simulink model "Simulation_2Sensors"  (R2020a)
settings: Solver=VariableStepAuto  StartTime=0.0  StopTime=18  RelTol=1e-3
values from neighbouring files (symbols this model uses):
  Pixels = [0 0 0 0 0 0 0 0 0 0 0 0 ... (1000000 elements, 1000x1000)]    [CrossMap.mat]    (also in GenerateCourseData.m = zeros(Height, Width); Pixels.mat = [0 0 0 0 0 0 0 0 0 0 0 0 ... (19600 elements, 140x140)])
  scale = 1    [GenerateCourseData.m]
undefined symbols (not defined in the file or in its folder): DiscIntNeverNeededParam, l, sensRange, w
libraries: simulink x1
settings Model: Creator=robot  LastModifiedBy=robot

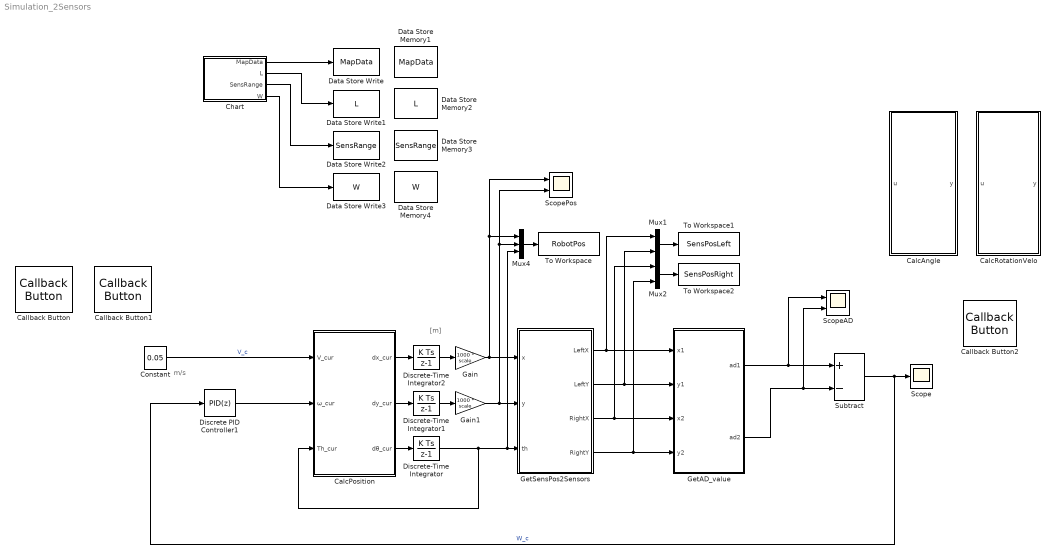
== system Simulation_2Sensors ==
  note: [m]
  note: m/s
  CalcAngle : MATLAB Function  TreatAsAtomicUnit=on
  CalcPosition : Subsystem
  CalcRotationVelo : MATLAB Function  TreatAsAtomicUnit=on
  Callback Button : CallbackButton  ButtonText=Generata Course Data
      settings: ClickFcn=run('GenerateCourseData.m')
  Callback Button1 : CallbackButton  ButtonText=Initialize
      settings: ClickFcn=run('init.m')
  Callback Button2 : CallbackButton  ButtonText=Animation Plot
      settings: ClickFcn=run('amimation.m')
  Chart : Stateflow chart  TreatAsAtomicUnit=on
  Constant : Constant  Value=0.05
  Data Store Memory1 : DataStoreMemory  DataStoreName=MapData  ReadBeforeWriteMsg=warning  WriteAfterWriteMsg=warning  WriteAfterReadMsg=warning  VectorParams1D=off  ShowAdditionalParam=off  OutDataTypeStr=double  Dimensions=[1000 ; 1000]
  Data Store Memory2 : DataStoreMemory  DataStoreName=L  ReadBeforeWriteMsg=warning  WriteAfterWriteMsg=warning  WriteAfterReadMsg=warning  VectorParams1D=off  ShowAdditionalParam=off  OutDataTypeStr=double  Dimensions=1
  Data Store Memory3 : DataStoreMemory  DataStoreName=SensRange  ReadBeforeWriteMsg=warning  WriteAfterWriteMsg=warning  WriteAfterReadMsg=warning  VectorParams1D=off  ShowAdditionalParam=off  OutDataTypeStr=double  Dimensions=1
  Data Store Memory4 : DataStoreMemory  DataStoreName=W  ReadBeforeWriteMsg=warning  WriteAfterWriteMsg=warning  WriteAfterReadMsg=warning  VectorParams1D=off  ShowAdditionalParam=off  OutDataTypeStr=double  Dimensions=1
  Data Store Write : DataStoreWrite  DataStoreName=MapData
  Data Store Write1 : DataStoreWrite  DataStoreName=L
  Data Store Write2 : DataStoreWrite  DataStoreName=SensRange
  Data Store Write3 : DataStoreWrite  DataStoreName=W
  Discrete PID Controller1 : simulink/Continuous/PID Controller  Controller=PID  Form=Parallel  TimeDomain=Discrete-time  UseExternalTs=off  SampleTime=-1  IntegratorMethod=Forward Euler  FilterMethod=Forward Euler  ControllerParametersSource=internal  P=1  I=0  D=0  UseFilter=on  N=100  TunerSelectOption=Transfer Function Based (PID Tuner App)  InitialConditionSource=internal  InitialConditionForIntegrator=0  InitialConditionForFilter=0  DifferentiatorICPrevScaledInput=0  ExternalReset=none  TrackingMode=off  Kt=1  LimitOutput=off  UpperSaturationLimit=inf  LowerSaturationLimit=-inf  LinearizeAsGain=off  AntiWindupMode=none  Kb=1  POutMin=[]  POutMax=[]  IOutMin=[]  IOutMax=[]  DOutMin=[]  DOutMax=[]  NOutMin=[]  NOutMax=[]  SumOutMin=[]  SumOutMax=[]  SaturationOutMin=[]  SaturationOutMax=[]  PParamMin=[]  PParamMax=[]  IParamMin=[]  IParamMax=[]  DParamMin=[]  DParamMax=[]  NParamMin=[]  NParamMax=[]  KbParamMin=[]  KbParamMax=[]  KtParamMin=[]  KtParamMax=[]  KbOutMin=[]  KbOutMax=[]  KtOutMin=[]  KtOutMax=[]  IntegratorOutMin=[]  IntegratorOutMax=[]  FilterOutMin=[]  FilterOutMax=[]  SumI1OutMin=[]  SumI1OutMax=[]  SumI2OutMin=[]  SumI2OutMax=[]  SumI3OutMin=[]  SumI3OutMax=[]  SumI4OutMin=[]  SumI4OutMax=[]  SumDOutMin=[]  SumDOutMax=[]  DifferentiatorOutMin=[]  DifferentiatorOutMax=[]  FilterDiffOutCoefMin=[]  FilterDiffOutCoefMax=[]  ReciprocalOutMin=[]  ReciprocalOutMax=[]  SumDenOutMin=[]  SumDenOutMax=[]  SumNumOutMin=[]  SumNumOutMax=[]  DivideOutMin=[]  DivideOutMax=[]  UdiffTsProdOutMin=[]  UdiffTsProdOutMax=[]  NTsProdOutMin=[]  NTsProdOutMax=[]  UintegralTsProdOutMin=[]  UintegralTsProdOutMax=[]  UngainTsProdOutMin=[]  UngainTsProdOutMax=[]  IntegratorContinuousStateAttributes=''  IntegratorStateMustResolveToSignalObject=off  IntegratorRTWStateStorageClass=Auto  FilterContinuousStateAttributes=''  FilterStateMustResolveToSignalObject=off  FilterRTWStateStorageClass=Auto  ParallelPVariant=InternalParameters  IdealPVariant=Disabled  IVariant=InternalParameters  DVariant=InternalParameters  IntegratorVariant=Discrete  SatVariant=Disabled  AWVariant=Passthrough  PCopyVariant=Disabled  TRVariant=Disabled  FdbkBlocksVariant=Forward  IdealPFdbkVariant=Disabled  SatFdbkVariant=Disabled  DerivativeFilterVariant=ForwardEulerFilter  NVariant=InternalParameters  NCopyVariant=Disabled  FilterICVariant=InternalICsFilter  IntegratorICVariant=InternalICs  ExternalResetVariant=Disabled  TRSumVariant=Passthrough  SumFdbkVariant=Disabled  SumVariant=Sum_PID  TsampFilterVariant=InternalTs  TsampNgainVariant=Passthrough  TsampIntegralVariant=Passthrough
  Discrete-Time Integrator : DiscreteIntegrator  InitialCondition=pi/6  SampleTime=-1  ICPrevOutput=DiscIntNeverNeededParam  ICPrevScaledInput=DiscIntNeverNeededParam
  Discrete-Time Integrator1 : DiscreteIntegrator  InitialCondition=0.3  SampleTime=-1  ICPrevOutput=DiscIntNeverNeededParam  ICPrevScaledInput=DiscIntNeverNeededParam
  Discrete-Time Integrator2 : DiscreteIntegrator  SampleTime=-1  ICPrevOutput=DiscIntNeverNeededParam  ICPrevScaledInput=DiscIntNeverNeededParam
  Gain : Gain  Gain=1000 * scale
  Gain1 : Gain  Gain=1000 * scale
  GetAD_value : MATLAB Function  TreatAsAtomicUnit=on
  GetSensPos2Sensors : MATLAB Function  TreatAsAtomicUnit=on
  Mux1 : Mux  Inputs=2
  Mux2 : Mux  Inputs=2
  Mux4 : Mux  Inputs=3
  Scope : Scope
  ScopeAD : Scope  NumInputPorts=2
  ScopePos : Scope  NumInputPorts=2
  Subtract : Sum  Inputs=+-
  To Workspace : ToWorkspace  VariableName=RobotPos  SampleTime=-1
  To Workspace1 : ToWorkspace  VariableName=SensPosLeft  SampleTime=-1
  To Workspace2 : ToWorkspace  VariableName=SensPosRight  SampleTime=-1
  wires:
  Constant/1 -> CalcPosition/1(V_cur)  "V_c"
  CalcPosition/3(dθ_cur) -> Discrete-Time Integrator/1
  Discrete-Time Integrator/1 -> CalcPosition/3(Th_cur), Mux4/3, GetSensPos2Sensors/3(th)
  GetSensPos2Sensors/1(LeftX) -> Mux1/1, GetAD_value/1(x1)
  GetSensPos2Sensors/2(LeftY) -> Mux1/2, GetAD_value/2(y1)
  Mux4/1 -> To Workspace/1
  Mux1/1 -> To Workspace1/1
  Mux2/1 -> To Workspace2/1
  GetSensPos2Sensors/3(RightX) -> Mux2/1, GetAD_value/3(x2)
  GetSensPos2Sensors/4(RightY) -> Mux2/2, GetAD_value/4(y2)
  GetAD_value/1(ad1) -> ScopeAD/1, Subtract/1
  GetAD_value/2(ad2) -> ScopeAD/2, Subtract/2
  Discrete-Time Integrator2/1 -> Gain/1
  Discrete-Time Integrator1/1 -> Gain1/1
  CalcPosition/1(dx_cur) -> Discrete-Time Integrator2/1
  CalcPosition/2(dy_cur) -> Discrete-Time Integrator1/1
  Gain/1 -> ScopePos/1, Mux4/1, GetSensPos2Sensors/1(x)
  Gain1/1 -> ScopePos/2, Mux4/2, GetSensPos2Sensors/2(y)
  Chart/1(MapData) -> Data Store Write/1
  Subtract/1 -> Discrete PID Controller1/1, Scope/1  "W_c"
  Chart/2(L) -> Data Store Write1/1
  Chart/3(SensRange) -> Data Store Write2/1
  Chart/4(W) -> Data Store Write3/1
  Discrete PID Controller1/1 -> CalcPosition/2(ω_cur)

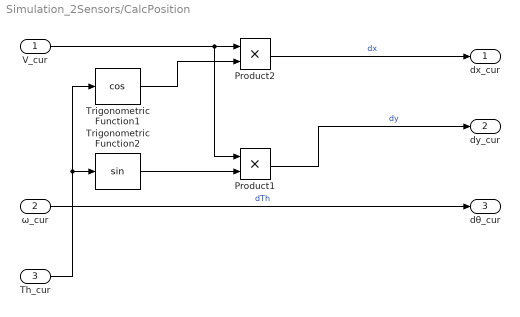
== system Simulation_2Sensors/CalcPosition ==
  V_cur : Inport
  ω_cur : Inport  Port=2
  Th_cur : Inport  Port=3
  Product1 : Product
  Product2 : Product
  Trigonometric Function1 : Trigonometry  Operator=cos
  Trigonometric Function2 : Trigonometry
  dx_cur : Outport  VectorParamsAs1DForOutWhenUnconnected=off
  dy_cur : Outport  Port=2  VectorParamsAs1DForOutWhenUnconnected=off
  dθ_cur : Outport  Port=3  VectorParamsAs1DForOutWhenUnconnected=off
  wires:
  V_cur/1 -> Product2/1, Product1/1
  Trigonometric Function1/1 -> Product2/2
  Th_cur/1 -> Trigonometric Function2/1, Trigonometric Function1/1
  Product2/1 -> dx_cur/1  "dx"
  Product1/1 -> dy_cur/1  "dy"
  Trigonometric Function2/1 -> Product1/2
  ω_cur/1 -> dθ_cur/1  "dTh"

== matlab function Simulation_2Sensors/CalcAngle ==
  data: u input; y output
function y = fcn(u)

y = u;

== matlab function Simulation_2Sensors/GetSensPos2Sensors ==
  data: x input; y input; th input; LeftX output; LeftY output; RightX output; RightY output; L data_store_memory; W data_store_memory
function [LeftX, LeftY, RightX, RightY] = fcn(x, y, th)
global L;
global W;

RobotParam.L = L; %[mm]
RobotParam.W = W;  %[mm]

SensOffset.Left = [RobotParam.L;
                   RobotParam.W];
            
SensOffset.Right = [RobotParam.L;
                    -RobotParam.W];

SensPos.Left = zeros(2, 1);
SensPos.Right = zeros(2, 1);

SensPos.Left = [x; y] + [cos(th), - sin(th) ; sin(th), cos(th)] * SensOffset.Left;
SensPos.Right = [x; y] + [cos(th), - sin(th) ; sin(th), cos(th)] * SensOffset.Right;

LeftX = SensPos.Left(1, 1);
LeftY = SensPos.Left(2, 1);

RightX = SensPos.Right(1, 1);
RightY = SensPos.Right(2, 1);

== matlab function Simulation_2Sensors/CalcRotationVelo ==
  data: u input; y output
function y = fcn(u)

y = u;

== matlab function Simulation_2Sensors/GetAD_value ==
  settings: updateMethod=DISCRETE
  data: x1 input; ad1 output; y1 input; x2 input; y2 input; ad2 output; MapData data_store_memory; SensRange data_store_memory
function [ad1, ad2] = fcn(x1, y1, x2, y2)
global SensRange;
global MapData

MaxNum_x = numel(MapData(1, :));
MaxNum_y = numel(MapData(:, 1));

Trimming1 = zeros(SensRange, SensRange);
Trimming2 = zeros(SensRange, SensRange);

for i = 1 : SensRange
    for j = 1 : SensRange  
        if (x1 - ceil(SensRange / 2) + j > 0) && (x1 + ceil(SensRange / 2) + j < MaxNum_x) && (y1 -ceil( SensRange / 2) + i > 0) && (y1 - ceil(SensRange / 2) + i < MaxNum_y)
            Trimming1(i, j) = MapData(ceil((x1 - SensRange / 2) + j), ceil((y1 - SensRange / 2) + i));
        else
            Trimming1(i, j) = NaN(1);
        end  
    end
end

for i = 1 : SensRange
    for j = 1 : SensRange  
        if (x2 - ceil(SensRange / 2) + j > 0) && (x2 + ceil(SensRange / 2) + j < MaxNum_x) && (y2 - ceil(SensRange / 2) + i > 0) && (y2 - ceil(SensRange / 2) + i < MaxNum_y)
            Trimming2(i, j) = MapData(ceil((x2 - SensRange / 2) + j), ceil((y2 - SensRange / 2) + i));
        else
            Trimming2(i, j) = NaN(1);
        end  
    end
end

ad1 = mean(Trimming1, 'all');
ad2 = mean(Trimming2, 'all');

end

== stateflow chart Simulation_2Sensors/Chart ==
  state GetMap
    entry:
    MapData = Pixels;
    L = l;
    W = w;
    SensRange = sensRange;
    flag = 1;
  state Idle
  (default) -> GetMap
  GetMap -> Idle : [flag == 1]
  data: Pixels parameter; MapData output; flag local; l parameter; sensRange parameter; w parameter; L output; SensRange output; W output
